simulink model "model"  (R2020b)
settings: Solver=VariableStepAuto  StartTime=0.0  StopTime=4  FixedStep=0.0001  RelTol=1e-3
undefined symbols (not defined in the file): b, J, K, Kd, Ki, Kp, L, R
settings Model: DataDictionary=motor_pos_data_dictionary.sldd  Creator=Arvind Hishikar  LastModifiedBy=Arvind Hishikar
settings SolverCC: MaxConsecutiveMinStep=10

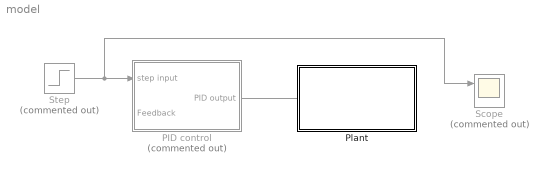
== system model ==
  PID control : Subsystem  Commented=on
  Plant : Subsystem
  Scope : Scope  Commented=on  NumInputPorts=2
  Step : Step  Commented=on  SampleTime=0
  wires:
  Step/1 -> Scope/1, PID control/1(step input)
  PID control/1(PID output) -> ?

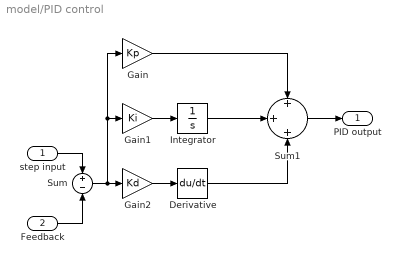
== system model/PID control ==
  step input : Inport
  Feedback : Inport  Port=2
  Derivative : Derivative
  Gain : Gain  Gain=Kp
  Gain1 : Gain  Gain=Ki
  Gain2 : Gain  Gain=Kd
  Integrator : Integrator
  Sum : Sum  Inputs=+|-
  Sum1 : Sum  Inputs=+||+||+
  PID output : Outport
  wires:
  Sum/1 -> Gain1/1, Gain/1, Gain2/1
  Derivative/1 -> Sum1/3
  Gain2/1 -> Derivative/1
  step input/1 -> Sum/1
  Gain/1 -> Sum1/1
  Feedback/1 -> Sum/2
  Sum1/1 -> PID output/1
  Gain1/1 -> Integrator/1
  Integrator/1 -> Sum1/2

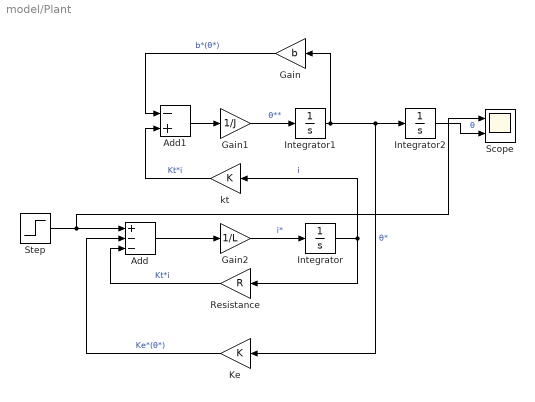
== system model/Plant ==
  Add : Sum  Inputs=+--
  Add1 : Sum  Inputs=-+
  Gain : Gain  Gain=b
  Gain1 : Gain  Gain=1/J
  Gain2 : Gain  Gain=1/L
  Integrator : Integrator
  Integrator1 : Integrator  UpperSaturationLimit=5  LowerSaturationLimit=-5
  Integrator2 : Integrator
  Ke : Gain  Gain=K
  Resistance : Gain  Gain=R
  Scope : Scope  NumInputPorts=2
  Step : Step  SampleTime=0
  kt : Gain  Gain=K
  wires:
  Integrator1/1 -> Gain/1, Ke/1, Integrator2/1  "θ*"
  Add/1 -> Gain2/1
  Gain1/1 -> Integrator1/1  "θ**"
  Integrator/1 -> Resistance/1, kt/1  "i"
  Gain/1 -> Add1/1  "b*(θ*)"
  Gain2/1 -> Integrator/1  "i*"
  Add1/1 -> Gain1/1
  Step/1 -> Scope/1, Add/1
  Resistance/1 -> Add/3  "Kt*i"
  kt/1 -> Add1/2  "Kt*i"
  Ke/1 -> Add/2  "Ke*(θ*)"
  Integrator2/1 -> Scope/2  "θ"
